simulink model "expansionTests"  (R2017b)
settings: Solver=FixedStepDiscrete  StartTime=0.0  StopTime=10.0  FixedStep=0.1  RelTol=1e-3
libraries: simulink x6
settings Model: Creator=cyarp  LastModifiedBy=cyarp

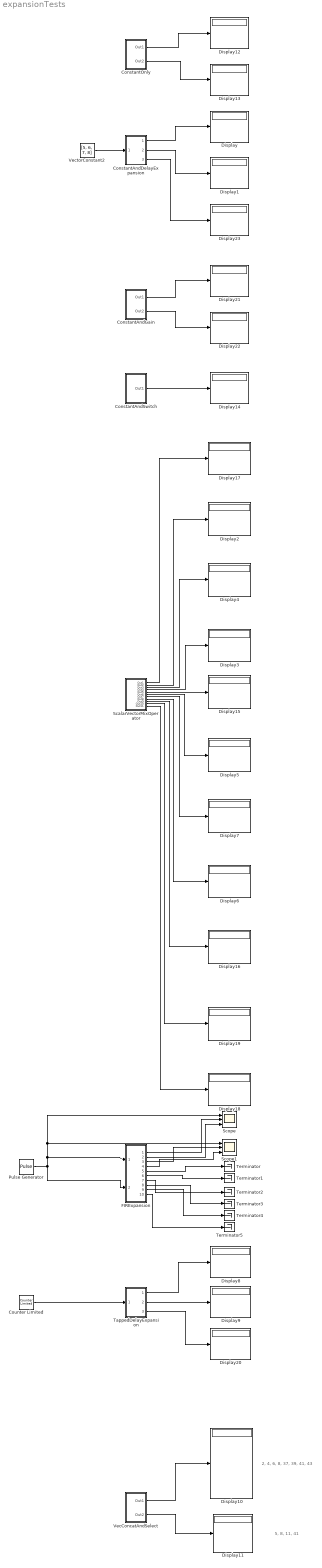
== system expansionTests ==
  note: 2, 4, 6, 8, 37, 39, 41, 43
  note: 5, 8, 11, 41
  ConstantAndDelayExpansion : Subsystem
  ConstantAndGain : Subsystem
  ConstantAndSwitch : Subsystem
  ConstantOnly : Subsystem
  Counter Limited : simulink/Sources/Counter Limited  uplimit=63  tsamp=0.1
  Display{,1..23} (24 alike) : Display
  FIRExpansion : Subsystem
  Pulse Generator : DiscretePulseGenerator  PulseType=Time based  Period=5  PulseWidth=50
  ScalarVectorMixOperator : Subsystem
  Scope : Scope  NumInputPorts=3
  Scope1 : Scope  NumInputPorts=3
  TappedDelayExpansion : Subsystem
  Terminator{,1..5} (6 alike) : Terminator
  VecConcatAndSelect : Subsystem
  VectorConstant2 : Constant  Value=[5, 6, 7, 8]
  wires:
  ConstantAndDelayExpansion/1(Out1) -> Display/1
  ConstantAndDelayExpansion/2(Out2) -> Display1/1
  ScalarVectorMixOperator/2(Out2) -> Display2/1
  ScalarVectorMixOperator/3(Out3) -> Display4/1
  ScalarVectorMixOperator/4(Out4) -> Display3/1
  ScalarVectorMixOperator/6(Out6) -> Display5/1
  ScalarVectorMixOperator/7(Out7) -> Display7/1
  ScalarVectorMixOperator/8(Out8) -> Display6/1
  Pulse Generator/1 -> Scope1/1, Scope/1, FIRExpansion/1(In1), FIRExpansion/2(In2)
  FIRExpansion/1(Out1) -> Scope/2
  FIRExpansion/2(Out2) -> Scope/3
  FIRExpansion/3(Out3) -> Scope1/2
  FIRExpansion/4(Out4) -> Scope1/3
  Counter Limited/1 -> TappedDelayExpansion/1(In1)
  TappedDelayExpansion/1(Out1) -> Display8/1
  TappedDelayExpansion/2(Out2) -> Display9/1
  VecConcatAndSelect/1(Out1) -> Display10/1
  VecConcatAndSelect/2(Out2) -> Display11/1
  ConstantOnly/1(Out1) -> Display12/1
  ConstantOnly/2(Out2) -> Display13/1
  ConstantAndSwitch/1(Out1) -> Display14/1
  ScalarVectorMixOperator/5(Out5) -> Display15/1
  ScalarVectorMixOperator/9(Out9) -> Display16/1
  ScalarVectorMixOperator/1(Out1) -> Display17/1
  ScalarVectorMixOperator/10(Out10) -> Display19/1
  ScalarVectorMixOperator/11(Out11) -> Display18/1
  TappedDelayExpansion/3(Out3) -> Display20/1
  ConstantAndGain/2(Out2) -> Display22/1
  ConstantAndGain/1(Out1) -> Display21/1
  FIRExpansion/5(Out5) -> Terminator/1
  FIRExpansion/6(Out6) -> Terminator1/1
  FIRExpansion/7(Out7) -> Terminator2/1
  FIRExpansion/8(Out8) -> Terminator3/1
  FIRExpansion/9(Out9) -> Terminator4/1
  FIRExpansion/10(Out10) -> Terminator5/1
  VectorConstant2/1 -> ConstantAndDelayExpansion/1(In1)
  ConstantAndDelayExpansion/3(Out3) -> Display23/1

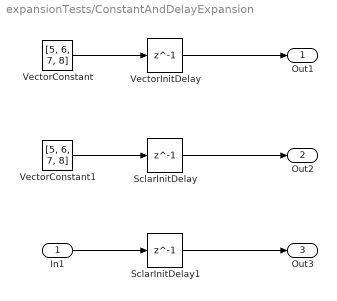
== system expansionTests/ConstantAndDelayExpansion ==
  In1 : Inport
  SclarInitDelay : Delay  DelayLength=1  InitialCondition=1
  SclarInitDelay1 : Delay  DelayLength=1  InitialCondition=1
  VectorConstant : Constant  Value=[5, 6, 7, 8]
  VectorConstant1 : Constant  Value=[5, 6, 7, 8]
  VectorInitDelay : Delay  DelayLength=1  InitialCondition=[1, 2, 3, 4]
  Out1 : Outport
  Out2 : Outport  Port=2
  Out3 : Outport  Port=3
  wires:
  VectorConstant/1 -> VectorInitDelay/1
  VectorInitDelay/1 -> Out1/1
  VectorConstant1/1 -> SclarInitDelay/1
  SclarInitDelay/1 -> Out2/1
  SclarInitDelay1/1 -> Out3/1
  In1/1 -> SclarInitDelay1/1

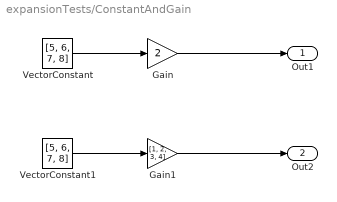
== system expansionTests/ConstantAndGain ==
  Gain : Gain  Gain=2
  Gain1 : Gain  Gain=[1, 2, 3, 4]
  VectorConstant : Constant  Value=[5, 6, 7, 8]
  VectorConstant1 : Constant  Value=[5, 6, 7, 8]
  Out1 : Outport
  Out2 : Outport  Port=2
  wires:
  VectorConstant/1 -> Gain/1
  Gain/1 -> Out1/1
  VectorConstant1/1 -> Gain1/1
  Gain1/1 -> Out2/1

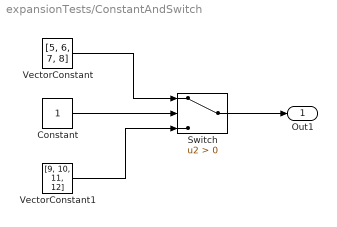
== system expansionTests/ConstantAndSwitch ==
  Constant : Constant
  Switch : Switch  Criteria=u2 > Threshold
  VectorConstant : Constant  Value=[5, 6, 7, 8]
  VectorConstant1 : Constant  Value=[9, 10, 11, 12]
  Out1 : Outport
  wires:
  Switch/1 -> Out1/1
  VectorConstant/1 -> Switch/1
  Constant/1 -> Switch/2
  VectorConstant1/1 -> Switch/3

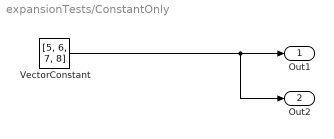
== system expansionTests/ConstantOnly ==
  VectorConstant : Constant  Value=[5, 6, 7, 8]
  Out1 : Outport
  Out2 : Outport  Port=2
  wires:
  VectorConstant/1 -> Out2/1, Out1/1

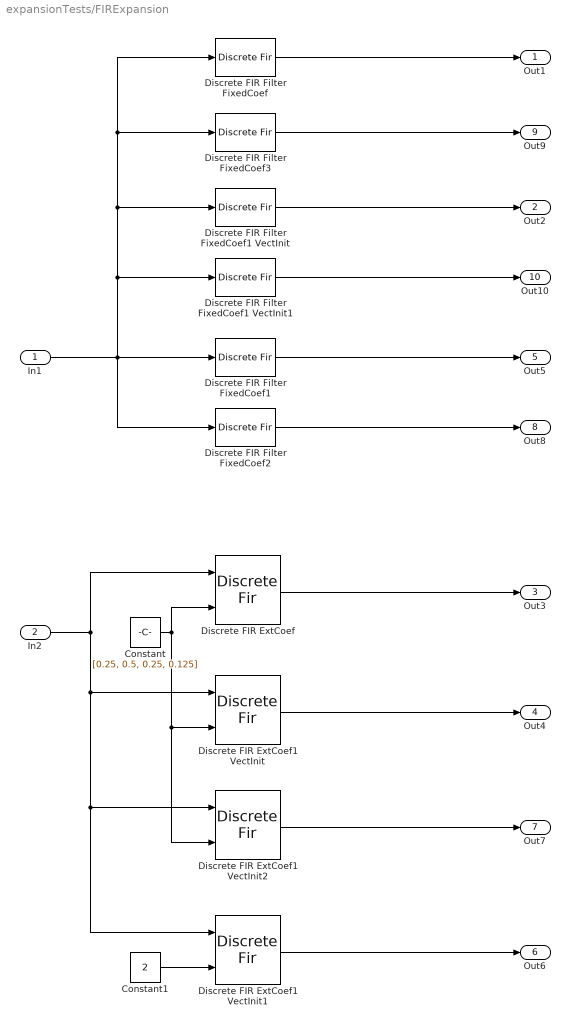
== system expansionTests/FIRExpansion ==
  In1 : Inport
  In2 : Inport  Port=2
  Constant : Constant  Value=[0.25, 0.5, 0.25, 0.125]
  Constant1 : Constant  Value=2
  Discrete FIR ExtCoef : DiscreteFir  CoefSource=Input port  Coefficients=[0.25, 0.5, 0.25, 0.125]
      settings: InputPortMap=u0,u1
  Discrete FIR ExtCoef1 VectInit : DiscreteFir  CoefSource=Input port  Coefficients=[0.25, 0.5, 0.25, 0.125]  InitialStates=[0, 0, 1]
      settings: InputPortMap=u0,u1
  Discrete FIR ExtCoef1 VectInit1 : DiscreteFir  CoefSource=Input port  Coefficients=[0.25, 0.5, 0.25, 0.125]
      settings: InputPortMap=u0,u1
  Discrete FIR ExtCoef1 VectInit2 : DiscreteFir  CoefSource=Input port  FilterStructure=Direct form transposed  Coefficients=[0.25, 0.5, 0.25, 0.125]  InitialStates=[0, 0, 1]
      settings: InputPortMap=u0,u1
  Discrete FIR Filter FixedCoef : DiscreteFir  FilterStructure=Direct form transposed  Coefficients=[0.25, 0.5, 0.25, 0.125]
  Discrete FIR Filter FixedCoef1 : DiscreteFir  FilterStructure=Direct form transposed  Coefficients=[2]
  Discrete FIR Filter FixedCoef1 VectInit : DiscreteFir  Coefficients=[0.25, 0.5, 0.25, 0.125]  InitialStates=[0, 0, 1]
  Discrete FIR Filter FixedCoef1 VectInit1 : DiscreteFir  Coefficients=[0.25, 0.5, 0.25, 0.125]  InitialStates=[0, 0, 1]  AccumDataTypeStr=Inherit: Same as product output
  Discrete FIR Filter FixedCoef2 : DiscreteFir  FilterStructure=Direct form transposed  Coefficients=[2]  OutDataTypeStr=Inherit: Same as input
  Discrete FIR Filter FixedCoef3 : DiscreteFir  FilterStructure=Direct form transposed  Coefficients=[0.25, 0.5, 0.25, 0.125]  OutDataTypeStr=Inherit: Same as input
  Out1 : Outport
  Out2 : Outport  Port=2
  Out3 : Outport  Port=3
  Out4 : Outport  Port=4
  Out5 : Outport  Port=5
  Out6 : Outport  Port=6
  Out7 : Outport  Port=7
  Out8 : Outport  Port=8
  Out9 : Outport  Port=9
  Out10 : Outport  Port=10
  wires:
  Discrete FIR Filter FixedCoef/1 -> Out1/1
  Constant/1 -> Discrete FIR ExtCoef/2, Discrete FIR ExtCoef1 VectInit2/2, Discrete FIR ExtCoef1 VectInit/2
  In1/1 -> Discrete FIR Filter FixedCoef2/1, Discrete FIR Filter FixedCoef1 VectInit1/1, Discrete FIR Filter FixedCoef3/1, Discrete FIR Filter FixedCoef/1, Discrete FIR Filter FixedCoef1 VectInit/1, Discrete FIR Filter FixedCoef1/1
  Discrete FIR ExtCoef1 VectInit/1 -> Out4/1
  Discrete FIR Filter FixedCoef1 VectInit/1 -> Out2/1
  Discrete FIR ExtCoef/1 -> Out3/1
  In2/1 -> Discrete FIR ExtCoef/1, Discrete FIR ExtCoef1 VectInit2/1, Discrete FIR ExtCoef1 VectInit1/1, Discrete FIR ExtCoef1 VectInit/1
  Discrete FIR Filter FixedCoef1/1 -> Out5/1
  Constant1/1 -> Discrete FIR ExtCoef1 VectInit1/2
  Discrete FIR ExtCoef1 VectInit1/1 -> Out6/1
  Discrete FIR ExtCoef1 VectInit2/1 -> Out7/1
  Discrete FIR Filter FixedCoef2/1 -> Out8/1
  Discrete FIR Filter FixedCoef3/1 -> Out9/1
  Discrete FIR Filter FixedCoef1 VectInit1/1 -> Out10/1

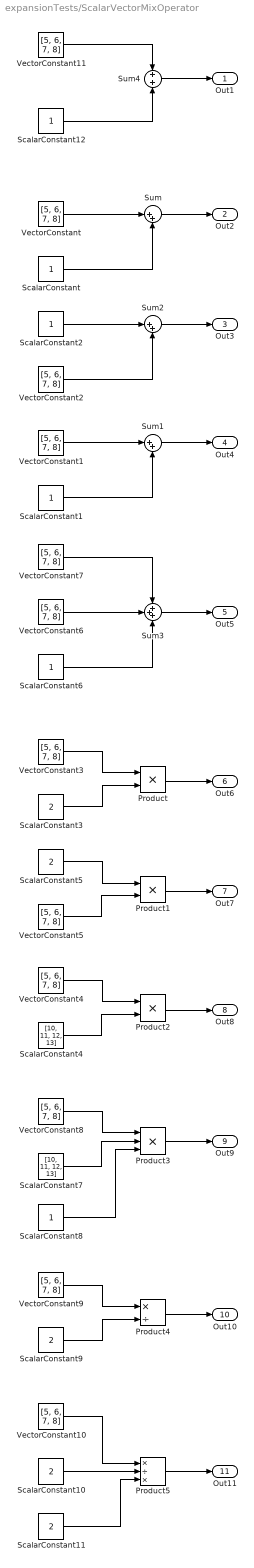
== system expansionTests/ScalarVectorMixOperator ==
  Product : Product
  Product1 : Product
  Product2 : Product
  Product3 : Product  Inputs=3
  Product4 : Product  Inputs=*/
  Product5 : Product  Inputs=*/*
  ScalarConstant{,1..2,6,8,12} (6 alike) : Constant
  ScalarConstant{3,5,9..11} (5 alike) : Constant  Value=2
  ScalarConstant4 : Constant  Value=[10, 11, 12, 13]
  ScalarConstant7 : Constant  Value=[10, 11, 12, 13]
  Sum : Sum  Inputs=|++
  Sum1 : Sum  Inputs=|++
  Sum2 : Sum  Inputs=|++
  Sum3 : Sum  Inputs=+++
  Sum4 : Sum  Inputs=2
  VectorConstant{,1..11} (12 alike) : Constant  Value=[5, 6, 7, 8]
  Out1 : Outport
  Out2 : Outport  Port=2
  Out3 : Outport  Port=3
  Out4 : Outport  Port=4
  Out5 : Outport  Port=5
  Out6 : Outport  Port=6
  Out7 : Outport  Port=7
  Out8 : Outport  Port=8
  Out9 : Outport  Port=9
  Out10 : Outport  Port=10
  Out11 : Outport  Port=11
  wires:
  ScalarConstant3/1 -> Product/2
  VectorConstant2/1 -> Sum2/2
  Sum2/1 -> Out3/1
  ScalarConstant2/1 -> Sum2/1
  Product/1 -> Out6/1
  ScalarConstant4/1 -> Product2/2
  Product1/1 -> Out7/1
  VectorConstant4/1 -> Product2/1
  VectorConstant/1 -> Sum/1
  ScalarConstant/1 -> Sum/2
  Product2/1 -> Out8/1
  VectorConstant3/1 -> Product/1
  Sum/1 -> Out2/1
  VectorConstant1/1 -> Sum1/1
  ScalarConstant1/1 -> Sum1/2
  ScalarConstant5/1 -> Product1/1
  VectorConstant5/1 -> Product1/2
  Sum1/1 -> Out4/1
  Sum3/1 -> Out5/1
  VectorConstant7/1 -> Sum3/1
  VectorConstant6/1 -> Sum3/2
  ScalarConstant6/1 -> Sum3/3
  ScalarConstant7/1 -> Product3/2
  VectorConstant8/1 -> Product3/1
  Product3/1 -> Out9/1
  ScalarConstant8/1 -> Product3/3
  VectorConstant9/1 -> Product4/1
  Product4/1 -> Out10/1
  ScalarConstant9/1 -> Product4/2
  Product5/1 -> Out11/1
  ScalarConstant10/1 -> Product5/2
  VectorConstant10/1 -> Product5/1
  ScalarConstant11/1 -> Product5/3
  VectorConstant11/1 -> Sum4/1
  ScalarConstant12/1 -> Sum4/2
  Sum4/1 -> Out1/1

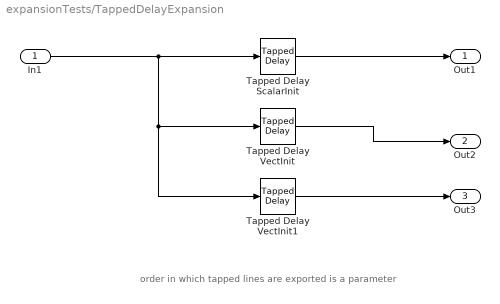
== system expansionTests/TappedDelayExpansion ==
  note: order in which tapped lines are exported is a parameter
  In1 : Inport
  Tapped Delay ScalarInit : simulink/Discrete/Tapped Delay  vinit=0.0  samptime=-1  NumDelays=4  DelayOrder=Oldest  includeCurrent=off
  Tapped Delay VectInit : simulink/Discrete/Tapped Delay  vinit=[1, 2, 3, 4]  samptime=-1  NumDelays=4  DelayOrder=Oldest  includeCurrent=off
  Tapped Delay VectInit1 : simulink/Discrete/Tapped Delay  vinit=1  samptime=-1  NumDelays=1  DelayOrder=Oldest  includeCurrent=off
  Out1 : Outport
  Out2 : Outport  Port=2
  Out3 : Outport  Port=3
  wires:
  Tapped Delay VectInit/1 -> Out2/1
  Tapped Delay ScalarInit/1 -> Out1/1
  In1/1 -> Tapped Delay VectInit1/1, Tapped Delay VectInit/1, Tapped Delay ScalarInit/1
  Tapped Delay VectInit1/1 -> Out3/1

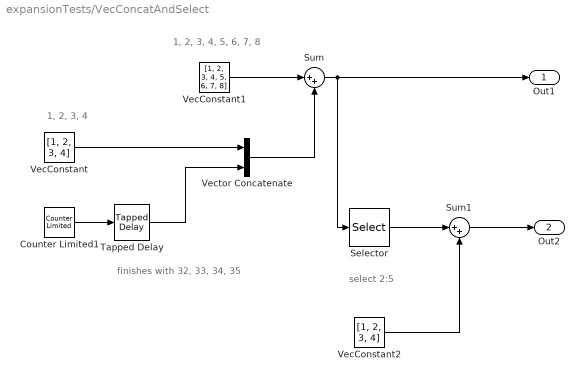
== system expansionTests/VecConcatAndSelect ==
  note: select 2:5
  note: 1, 2, 3, 4, 5, 6, 7, 8
  note: 1, 2, 3, 4
  note: finishes with 32, 33, 34, 35
  Counter Limited1 : simulink/Sources/Counter Limited  uplimit=63  tsamp=0.1
  Selector : Selector  InputPortWidth=8  IndexOptions=Index vector (dialog)  Indices=[2:5]  OutputSizes=1
  Sum : Sum  Inputs=|++
  Sum1 : Sum  Inputs=|++
  Tapped Delay : simulink/Discrete/Tapped Delay  vinit=0.0  samptime=-1  NumDelays=4  DelayOrder=Oldest  includeCurrent=off
  VecConstant : Constant  Value=[1, 2, 3, 4]  OutDataTypeStr=uint8
  VecConstant1 : Constant  Value=[1, 2, 3, 4, 5, 6, 7, 8]  OutDataTypeStr=uint8
  VecConstant2 : Constant  Value=[1, 2, 3, 4]  OutDataTypeStr=uint8
  Vector Concatenate : Concatenate
  Out1 : Outport
  Out2 : Outport  Port=2
  wires:
  Counter Limited1/1 -> Tapped Delay/1
  Sum1/1 -> Out2/1
  VecConstant1/1 -> Sum/1
  VecConstant2/1 -> Sum1/2
  Tapped Delay/1 -> Vector Concatenate/2
  Selector/1 -> Sum1/1
  Sum/1 -> Out1/1, Selector/1
  Vector Concatenate/1 -> Sum/2
  VecConstant/1 -> Vector Concatenate/1
